simulink model "problem1"  (R2013a)
settings: Solver=ode14x  StartTime=0.0  StopTime=10.0  FixedStep=0.0001  RelTol=1e-3
libraries: simulink x1
settings Model: Creator=Samanth  LastModifiedBy=Samanth
settings SolverCC: ShapePreserveControl=EnableAll

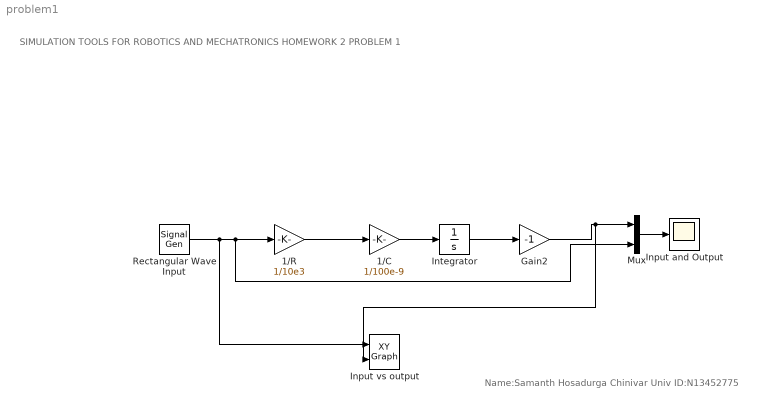
== system problem1 ==
  note: Name:Samanth Hosadurga Chinivar
      | Univ ID:N13452775
  note: SIMULATION TOOLS FOR ROBOTICS AND MECHATRONICS
      |
      |                                                                                                               HOMEWORK 2
      |                                                                                                              PROBLEM 1
  1/C : Gain  Gain=1/100e-9
  1/R : Gain  Gain=1/10e3
  Gain2 : Gain  Gain=-1
  Input and Output : Scope
      settings: YMin=-1  YMax=13
  Input vs output : simulink/Sinks/XY Graph  xmin=-1  xmax=3  ymin=0  ymax=15  st=-1
  Integrator : Integrator
  Mux : Mux  Inputs=2
  Rectangular Wave Input : SignalGenerator  WaveForm=square  Frequency=40
  wires:
  1/R/1 -> 1/C/1
  1/C/1 -> Integrator/1
  Integrator/1 -> Gain2/1
  Gain2/1 -> Input vs output/2, Mux/1
  Mux/1 -> Input and Output/1
  Rectangular Wave Input/1 -> Input vs output/1, Mux/2, 1/R/1
